simulink model "stateflow_functions"  (R2015b)
settings: Solver=VariableStepAuto  StartTime=0.0  StopTime=10.0  RelTol=1e-3
settings Model: Creator=ladmin  LastModifiedBy=ladmin

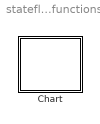
== system stateflow_functions ==
  Chart : Stateflow chart  TreatAsAtomicUnit=on

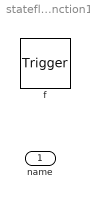
== system stateflow_functions/Chart/function1 ==
  name : Inport  OutDataTypeStr=double  PortDimensions=1
  f : TriggerPort  TriggerType=function-call
      settings: CopyFcn=Stateflow.SLINSF.SimulinkMan.removeBlockPreDeleteFcn  PreDeleteFcn=Stateflow.SLINSF.SimulinkMan.unsafePredeleteFcn

== stateflow chart stateflow_functions/Chart ==
  state function1(name) [function]
  state graphical(without,subchart) [function]
  state graphical1(with,subchart) [function]
    state ABC
  data: name function_input double size=1; without function_input; subchart function_input; with function_input; subchart function_input; name function_input
  function function(name):
    | function function(name)
